simulink model "RTOS_Mail_blocking_Blinky"  (R2020a)
settings: Solver=FixedStepDiscrete  StartTime=0.0  StopTime=10.0  FixedStep=1e-3  RelTol=1e-3
libraries: mbed_lib x6
settings Model: MbedPath=E:\GitSynology\mbed_target\targets\NUCLEO_F303RE  Creator=oh  LastModifiedBy=oh
settings DataIOCC: LimitDataPoints=on  SaveFormat=Array  ReturnWorkspaceOutputs=off
settings OptimizationCC: DefaultParameterBehavior=Inlined  EnhancedBackFolding=on  PassReuseOutputArgsAs=Individual arguments  ZeroExternalMemoryAtStartup=off  ZeroInternalMemoryAtStartup=off  OptimizeBlockOrder=speed  DifferentSizesBufferReuse=on  OptimizationCustomize=off  EfficientTunableParamExpr=on
settings DebuggingCC: SolverPrmCheckMsg=warning  ParameterTunabilityLossMsg=error  SFUnexpectedBacktrackingDiag=warning  SFNoUnconditionalDefaultTransitionDiag=warning  SFExecutionAtInitializationDiag=none  ArithmeticOperatorsInVariantConditions=warning
settings HardwareCC: ProdBitPerPointer=32  ProdBitPerSizeT=32  ProdBitPerPtrDiffT=32  ProdLargestAtomicInteger=Long  ProdLargestAtomicFloat=Double  ProdWordSize=32  ProdHWDeviceType=ARM Compatible->ARM Cortex
settings ModelReferenceCC: PropagateSignalLabelsOutOfModel=off
settings SFSimCC: SimUseLocalCustomCode=off  MATLABDynamicMemAlloc=off  CustomCodeUndefinedFunction=UseInterfaceOnly
settings RTWCC: Description=MbedTarget (Embedded Target for Embedded Coder)  SystemTargetFile=mbed_ert.tlc  TemplateMakefile=mbed_ert.tmf  RTWUseLocalCustomCode=off  TargetLang=C++
settings CodeAppCC: ForceParamTrailComments=on  IgnoreCustomStorageClasses=off  OperatorAnnotations=on  SimulinkDataObjDesc=on  SFDataObjDesc=on  InsertBlockDesc=on
settings STFCustomTargetCC: TargetLibSuffix=.a  MultiwordLength=256  GenerateSampleERTMain=on  CombineOutputUpdateFcns=on  ERTCustomFileBanners=on  SupportContinuousTime=off  SupportNonInlinedSFcns=off  RemoveResetFunc=on  MATLABClassNameForMDSCustomization=Simulink.SoftwareTarget.ERTCustomization  ModelStepFunctionPrototypeControlCompliant=on  SystemTargetFile=mbed_ert.tlc
settings ERTTargetCC: GenerateSampleERTMain=on  ParMdlRefBuildCompliant=off  CompOptLevelCompliant=off  ConcurrentExecutionCompliant=off  CPPClassGenCompliant=off  UseToolchainInfoCompliant=off  InlinedParameterPlacement=NonHierarchical  ERTCustomFileTemplate=mbed_ert_file_process.tlc
settings ConfigComp: CovMetricSettings=dw  CovHtmlReporting=on  CovSaveCumulativeToWorkspaceVar=on  CovSaveSingleToWorkspaceVar=on  CovExternalEMLEnable=off  CovSFcnEnable=off

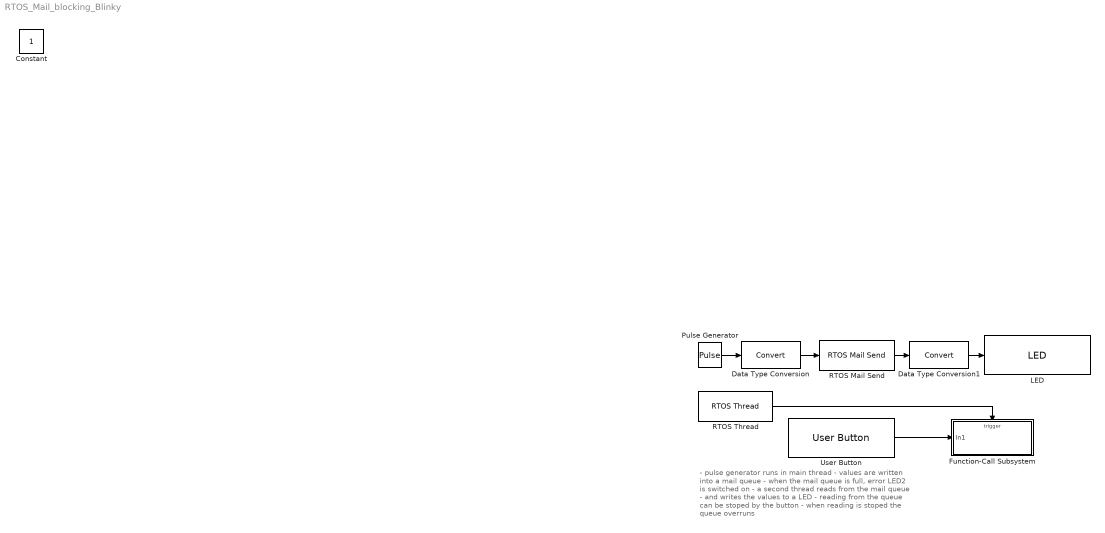
== system RTOS_Mail_blocking_Blinky ==
  note: - pulse generator runs in main thread
      | - values are written into a mail queue
      | - when the mail queue is full, error LED2 is switched on
      | - a second thread reads from the mail queue
      | - and writes the values to a LED
      | - reading from the queue can be stoped by the button
      | - when reading is stoped the queue overruns
  Data Type Conversion : DataTypeConversion
  Data Type Conversion1 : DataTypeConversion
  Function-Call Subsystem : Subsystem  TreatAsAtomicUnit=on
  LED : mbed_lib/GPIO/LED  nLED=2  SampleTime=-1
      settings: SourceProductName=Mbed Target
  Pulse Generator : DiscretePulseGenerator  PulseType=Time based  Period=1  PulseWidth=20
  RTOS Mail Send : mbed_lib/RTOS/RTOS Mail Send  MailNumber=1  Timeout=1000  Depth=50  NumElements=1  DataType=uint8  EnableError=on
      settings: SourceProductName=Mbed Target
  RTOS Thread : mbed_lib/RTOS/RTOS Thread  ThreadPriority=Normal  StackOption=Default  StackSize=0  Timing=0
      settings: SourceProductName=Mbed Target
  User Button : mbed_lib/GPIO/User Button  SampleTime=0.1
      settings: SourceProductName=Mbed Target
  Constant : Constant  IOType=siggen
  wires:
  Pulse Generator/1 -> Data Type Conversion/1
  Data Type Conversion/1 -> RTOS Mail Send/1
  RTOS Mail Send/1 -> Data Type Conversion1/1
  Data Type Conversion1/1 -> LED/1
  RTOS Thread/1 -> Function-Call Subsystem/Trigger
  User Button/1 -> Function-Call Subsystem/1(In1)

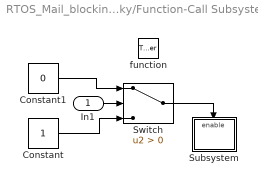
== system RTOS_Mail_blocking_Blinky/Function-Call Subsystem ==
  In1 : Inport
  function : TriggerPort  TriggerType=function-call  VariantControl=Variant
  Constant : Constant
  Constant1 : Constant  Value=0
  Subsystem : Subsystem
  Switch : Switch  Criteria=u2 > Threshold
  wires:
  In1/1 -> Switch/2
  Switch/1 -> Subsystem/Enable
  Constant1/1 -> Switch/1
  Constant/1 -> Switch/3

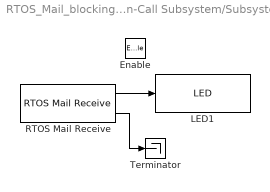
== system RTOS_Mail_blocking_Blinky/Function-Call Subsystem/Subsystem ==
  Enable : EnablePort
  LED1 : mbed_lib/GPIO/LED  nLED=1  SampleTime=-1
      settings: SourceProductName=Mbed Target
  RTOS Mail Receive : mbed_lib/RTOS/RTOS Mail Receive  MailNumber=1  Timeout=4294967295  NumElements=1  DataType=uint8
      settings: SourceProductName=Mbed Target
  Terminator : Terminator
  wires:
  RTOS Mail Receive/1 -> LED1/1
  RTOS Mail Receive/2 -> Terminator/1
